simulink model "WESDem_SetPoint"  (R2016b)
settings: configuration reference "CodeGenConfigSet" (kept outside this file)
values from neighbouring files (symbols this model uses):
  EISGov_st3valid_C = Calibration.Parameter    [init_WESDem_SetPoint.m]
  WESDem_dnAcc0_C = Calibration.Parameter    [init_WESDem_SetPoint.m]
  WESDem_dnAcc1_C = Calibration.Parameter    [init_WESDem_SetPoint.m]
  WESDem_dnAcc3_C = Calibration.Parameter    [init_WESDem_SetPoint.m]
  WESDem_dnDecn0_C = Calibration.Parameter    [init_WESDem_SetPoint.m]
  WESDem_dnDecn1_C = Calibration.Parameter    [init_WESDem_SetPoint.m]
  WESDem_dnDecn2_C = Calibration.Parameter    [init_WESDem_SetPoint.m]
  WESDem_nDelta_C = Calibration.Parameter    [init_WESDem_SetPoint.m]
  WESDem_nMin0_C = Calibration.Parameter    [init_WESDem_SetPoint.m]
  WESDem_nMin1_C = Calibration.Parameter    [init_WESDem_SetPoint.m]
  WESDem_nMin2_C = Calibration.Parameter    [init_WESDem_SetPoint.m]
  WESDem_nMin3_C = Calibration.Parameter    [init_WESDem_SetPoint.m]
  WESDem_nMode0_C = Calibration.Parameter    [init_WESDem_SetPoint.m]
  WESDem_nMode1_C = Calibration.Parameter    [init_WESDem_SetPoint.m]
  WESDem_nMode2_C = Calibration.Parameter    [init_WESDem_SetPoint.m]
  WESDem_nMode3_C = Calibration.Parameter    [init_WESDem_SetPoint.m]
  WESDem_nSetPHi0_C = Calibration.Parameter    [init_WESDem_SetPoint.m]
  WESDem_nSetPHi1_C = Calibration.Parameter    [init_WESDem_SetPoint.m]
  WESDem_nSetPHi2_C = Calibration.Parameter    [init_WESDem_SetPoint.m]
  WESDem_nSetPHi3_C = Calibration.Parameter    [init_WESDem_SetPoint.m]
  WESDem_nTipStp_C = Calibration.Parameter    [init_WESDem_SetPoint.m]
  WESDem_rAPPThresFrzI_C = Calibration.Parameter    [init_WESDem_SetPoint.m]
  WESDem_SetPLoTipInRmpSlopeNeg_C = Calibration.Parameter    [init_WESDem_SetPoint.m]
  WESDem_SetPLoTipInRmpSlopePos_C = Calibration.Parameter    [init_WESDem_SetPoint.m]
  WESDem_stASDrfInit_C = Calibration.Parameter    [init_WESDem_SetPoint.m]
  WESDem_stCurr_C = Calibration.Parameter    [init_WESDem_SetPoint.m]
  WESDem_stCurrvalid_C = Calibration.Parameter    [init_WESDem_SetPoint.m]
  WESDem_stMskFrzRls_C = Calibration.Parameter    [init_WESDem_SetPoint.m]
  WESDem_swtTrqHiSel_C = Calibration.Parameter    [init_WESDem_SetPoint.m]
  WESDem_swtTrqLoSel_C = Calibration.Parameter    [init_WESDem_SetPoint.m]
  WESDem_tiPT1_C = Calibration.Parameter    [init_WESDem_SetPoint.m]
  WESDem_tiTrqHiPT1_C = Calibration.Parameter    [init_WESDem_SetPoint.m]
  WESDem_tiTrqLoPT1_C = Calibration.Parameter    [init_WESDem_SetPoint.m]
undefined symbols (not defined in the file or in its folder): CruiseCtl_State_conv, Switch_conv, WESDem_SetPoint_DT, WESDem_State_conv
libraries: CXLib x23, simulink x15
(part 1 of 2)
settings Model: Creator=zhoukai  LastModifiedBy=zhoukai
settings ConfigSetRef: SourceLocation=Base Workspace

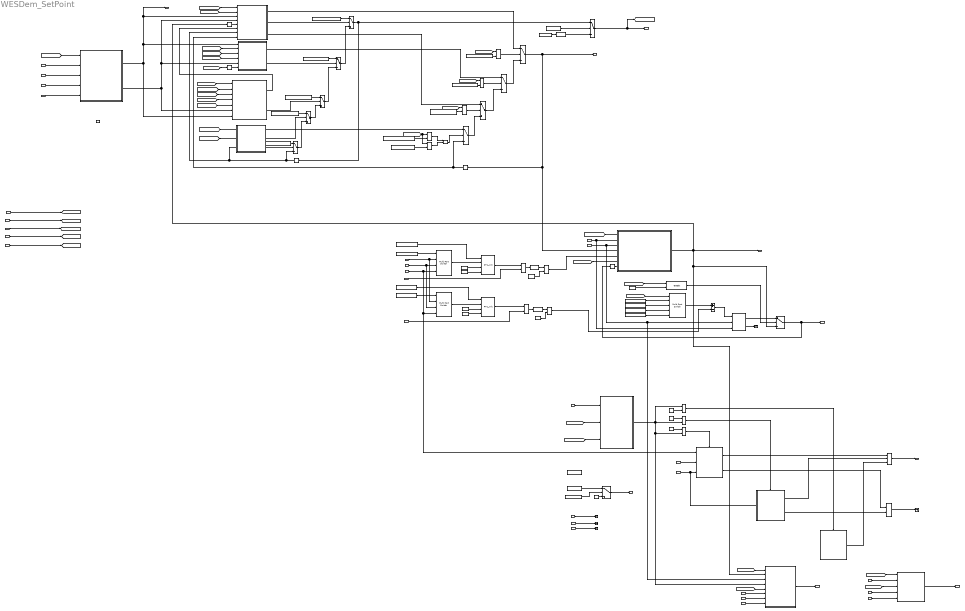
== system WESDem_SetPoint ==
  APP_r : Inport  Tag=%  Description=Acceleration pedal sensor 1 value after fault handling  OutMin=0  OutMax=100  OutDataTypeStr=Accpedal_rate
  CoETS_trqInrSetSlow : Inport  Tag=Nm  Description=Filtered inner torque ( positive torque) desired value (standard signal path) generated out of CoPT_trqDesEng  Port=2  OutMin=-3276  OutMax=3276  OutDataTypeStr=Trq_Nm
  CrCtl_st : Inport  Description=Application parameter for Cruise Control state  Port=3  OutDataTypeStr=Enum: CruiseCtl_State_conv
  DrvDem_swtDrvNGovActv : Inport  Description=Switch to activate DrvDem  Port=4  OutDataTypeStr=Enum: Switch_conv
  GlbDa_stTrqDem : Inport  Description=Contains highest prior function with torque demand  Port=5  OutMin=0  OutMax=4294967295  OutDataTypeStr=State_uint32
  HLSDem_nSetPHi : Inport  Tag=rpm  Description=Maximum engine speed of HLSDem  Port=6  OutMin=0  OutMax=6000  OutDataTypeStr=EngSpeed_rpm
  HLSDem_nSetPLo : Inport  Tag=rpm  Description=Minimum engine speed of HLSDem  Port=7  OutMin=0  OutMax=6000  OutDataTypeStr=EngSpeed_rpm
  MoFPTO_nMax0CalMsgA : Inport  Tag=rpm  Description=MoFPTO_nMaxCalMsgA[0]  Port=8  OutMin=0  OutMax=6000  OutDataTypeStr=EngSpeed_rpm
  MoFPTO_nMax1CalMsgA : Inport  Tag=rpm  Description=MoFPTO_nMaxCalMsgA[1]  Port=9  OutMin=0  OutMax=6000  OutDataTypeStr=EngSpeed_rpm
  MoFPTO_nMax2CalMsgA : Inport  Tag=rpm  Description=MoFPTO_nMaxCalMsgA[2]  Port=10  OutMin=0  OutMax=6000  OutDataTypeStr=EngSpeed_rpm
  MoFPTO_nMax3CalMsgA : Inport  Tag=rpm  Description=MoFPTO_nMaxCalMsgA[3]  Port=11  OutMin=0  OutMax=6000  OutDataTypeStr=EngSpeed_rpm
  PthLead_trqInrCurr : Inport  Tag=Nm  Description=Actual percent engine torque  Port=12  OutMin=-3000  OutMax=3000  OutDataTypeStr=Trq_Nm
  PthLead_trqInrLead : Inport  Tag=Nm  Description=Inner torque lead value  Port=13  OutMin=-3000  OutMax=3000  OutDataTypeStr=Trq_Nm
  PthSet_trqInrSet : Inport  Tag=Nm  Description=Inner torque set value after monitoring limitation  Port=14  OutMin=-3000  OutMax=3276.7  OutDataTypeStr=Trq_Nm
  VehV_v : Inport  Tag=km/h  Description=Vehicle speed  Port=15  OutMin=0  OutMax=250  OutDataTypeStr=VehSpeed_km_h
  WESDem_stCfg : Inport  Description=Configuration of the actual operating mode  Port=16  OutMin=0  OutMax=65535  OutDataTypeStr=State_uint16
  WESDem_stCrCtl : Inport  Description=State control of the working engine speed demand  Port=17  OutMin=0  OutMax=65535  OutDataTypeStr=State_uint16
  WESDem_stMode : Inport  Description=Operating mode of the working engine speed demand  Port=18  OutMin=0  OutMax=255  OutDataTypeStr=State_uint8
  WESDem_stModeChange : Inport  Description=Operating mode change of the working engine speed demand  Port=19  OutMin=0  OutMax=255  OutDataTypeStr=State_uint8
  Epm_nEng : Inport  Tag=rpm  Description=Engine speed  Port=20  OutMin=0  OutMax=6000  OutDataTypeStr=EngSpeed_rpm
  WESDem_facFdbkLo : Inport  Tag=rpm/Nm  Description=Feedback factor for the lower setpoint  Port=21  OutMin=-20  OutMax=20  OutDataTypeStr=FdbkNm2rpm_rpm_Nm
  WESDem_facFdbkHi : Inport  Tag=rpm/Nm  Description=Feedback factor for the higher setpoint  Port=22  OutMin=-20  OutMax=20  OutDataTypeStr=FdbkNm2rpm_rpm_Nm
  WESDem_stStrtBtnSP : Inport  Description=Status of working engine speed setpoint through start button  Port=23  OutMin=0  OutMax=255  OutDataTypeStr=State_uint8
  WESDem_nStrtBtnSP : Inport  Tag=rpm  Description=Working engine speed setpoint through start button  Port=24  OutMin=0  OutMax=6000  OutDataTypeStr=EngSpeed_rpm
  WESDem_stEISGovCfg : Inport  Description=Status of configuration of the EISGov structure  Port=25  OutMin=0  OutMax=255  OutDataTypeStr=State_uint8
  WESDem_vMaxActv : Inport  Tag=km/h  Description=Vehicle speed threshold for activation of the WESDem  Port=26  OutMin=0  OutMax=255  OutDataTypeStr=VehSpeed_km_h
  Asdrf_stInitin : Inport  Description=Status of Initialisation of ASD reference filter  Port=27  OutMin=0  OutMax=255  OutDataTypeStr=State_uint8
  WESDem_stShutOff : Inport  Description=Shut off conditions for the Working engine speed Demand  Port=28  OutMin=0  OutMax=65535  OutDataTypeStr=State_uint16
  function : TriggerPort  TriggerType=function-call  VariantControl=Variant
  ActionToNoInit : Subsystem
  Constant : Constant  Value=WESDem_State_conv.WESDEM_STOFFRAMP  OutDataTypeStr=Inherit: Inherit via back propagation
  Constant1 : Constant  Value=WESDem_swtTrqLoSel_C
  Constant10 : Constant  Value=WESDem_tiTrqHiPT1_C
  Constant11 : Constant  Value=WESDem_State_conv.WESDEM_STNEUTRAL  OutDataTypeStr=Inherit: Inherit via back propagation
  Constant{2..5,12,14,31} (7 alike) : Constant  Value=0  OutDataTypeStr=Inherit: Inherit via back propagation
  Constant13 : Constant  Value=7  OutDataTypeStr=Inherit: Inherit via back propagation
  Constant15 : Constant  Value=WESDem_nSetPHi0_C
  Constant16 : Constant  Value=WESDem_nSetPHi1_C
  Constant17 : Constant  Value=WESDem_nSetPHi2_C
  Constant18 : Constant  Value=WESDem_nSetPHi3_C
  Constant19 : Constant  Value=WESDem_State_conv.WESDEM_STOFF  OutDataTypeStr=Inherit: Inherit via back propagation
  Constant20 : Constant  Value=WESDem_State_conv.WESDEM_STOFFRAMP  OutDataTypeStr=Inherit: Inherit via back propagation
  Constant21 : Constant  Value=WESDem_stCurr_C
  Constant22 : Constant  Value=WESDem_stCurrvalid_C
  Constant23 : Constant  Value=EISGov_st3valid_C
  Constant24 : Constant  Value=WESDem_State_conv.WESDEM_STOFF  OutDataTypeStr=Inherit: Inherit via back propagation
  Constant25 : Constant  Value=WESDem_State_conv.WESDEM_STRESRAMP  OutDataTypeStr=Inherit: Inherit via back propagation
  Constant26 : Constant  Value=WESDem_State_conv.WESDEM_STACCDEC  OutDataTypeStr=Inherit: Inherit via back propagation
  Constant27 : Constant  Value=WESDem_State_conv.WESDEM_STNEUTRAL  OutDataTypeStr=Inherit: Inherit via back propagation
  Constant28 : Constant  Value=0
  Constant29 : Constant
  Constant30 : Constant  Value=2
  Constant6 : Constant  Value=WESDem_State_conv.WESDEM_STRESRAMP  OutDataTypeStr=Inherit: Inherit via back propagation
  Constant7 : Constant  Value=WESDem_swtTrqHiSel_C
  Constant8 : Constant  Value=WESDem_State_conv.WESDEM_STACCDEC  OutDataTypeStr=Inherit: Inherit via back propagation
  Constant9 : Constant  Value=WESDem_tiTrqLoPT1_C
  Data Store Memory : DataStoreMemory  DataStoreName=EISGov_st3  ReadBeforeWriteMsg=warning  WriteAfterWriteMsg=warning  WriteAfterReadMsg=warning  ShowAdditionalParam=off
  Data Store Read : DataStoreRead  DataStoreName=EISGov_st3
  Data Type Conversion : DataTypeConversion
  Data Type Conversion1 : DataTypeConversion
  Data Type Conversion2 : DataTypeConversion
  Delay : Delay  DelayLength=1  InitialCondition=WESDem_State_conv.WESDEM_STOFF
  Delay2 : Delay  DelayLength=1  InitialCondition=0
  Delay3 : Delay  DelayLength=1
  Delay4 : Delay  DelayLength=1
  Delay5 : Delay  DelayLength=1  InitialCondition=WESDem_State_conv.WESDEM_STOFF
  EISGov initialization : Subsystem
  GetBit1 : CXLib/GetBit  dataTypeString=uint16  dataLength=0
      settings: AttributesFormatString=Get bit from %<dataTypeString>
  Interface to the EISGov : Subsystem
  Logical Operator1 : Logic  Operator=OR  AllPortsSameDT=off  OutDataTypeStr=boolean
  Merge : Merge  Inputs=3
  Merge1 : Merge
  MinMax : MinMax  Function=max  Inputs=2
  MinMax1 : MinMax  Function=max  Inputs=2
  Multiport Switch : MultiPortSwitch  DataPortOrder=Zero-based contiguous
  Multiport Switch1 : MultiPortSwitch  DataPortOrder=Zero-based contiguous
  Multiport Switch2 : MultiPortSwitch  DataPortOrder=Zero-based contiguous  Inputs=4
  "Normal operation " : Subsystem  TreatAsAtomicUnit=on
  PT1_Init : CXLib/PT1_Init
  PT1_Init1 : CXLib/PT1_Init
  Product : Product
  Product1 : Product
  Relational Operator{3..10} (8 alike) : RelationalOperator  Operator===  OutDataTypeStr=boolean  RndMeth=Simplest
  Saturation_S1 : CXLib/Saturation_S16
  Subsystem1 : Subsystem
  Subsystem2 : Subsystem
  Subtract1 : Sum  Inputs=+-
  Switch{1..12} (12 alike) : Switch  Criteria=u2 ~= 0
  Terminator{,1..4} (5 alike) : Terminator
  WESDem_OffInit : Subsystem
  WESDem_OnInit : Subsystem
  WESDem_stCrCtl001 : Subsystem
  "WESDem_stCrCtl002 " : Subsystem
  WESDem_stCrCtl004 : Subsystem
  WESDem_stCrCtl007 : Subsystem
  WESDem_nMax : Outport  Tag=rpm  Description=maximum engine speed in selected mode  OutMin=0  OutMax=6000  OutDataTypeStr=EngSpeed_rpm
  WESDem_nSetPHi : Outport  Tag=rpm  Description=Higher setpoint speed interval of WESDem  Port=2  OutMin=0  OutMax=6000  OutDataTypeStr=EngSpeed_rpm
  WESDem_nSetPLo : Outport  Tag=rpm  Description=Lower setpoint speed interval of WESDem  Port=3  OutMin=0  OutMax=6000  OutDataTypeStr=EngSpeed_rpm
  WESDem_stActvReq : Outport  Description=WESDem activation request for EISGov  Port=4  OutMin=0  OutMax=1  OutDataTypeStr=boolean
  WESDem_stCrCtlShutOff : Outport  Description=Shut off of the cruise control  Port=5  OutMin=0  OutMax=1  OutDataTypeStr=boolean
  WESDem_stCurr : Outport  Description=Status of the working engine Speed Control  Port=6  OutDataTypeStr=Enum: WESDem_State_conv
  WESDem_trqReq : Outport  Tag=Nm  Description=Torque intialization request of working engine speed demand  Port=7  OutMin=-3276  OutMax=3276  OutDataTypeStr=Trq_Nm
  WESDem_nPrelimSetP_mp : Outport  Tag=rpm  Description=Engine speed set point before access by external engine speed  Port=8  OutMin=0  OutMax=6000  OutDataTypeStr=EngSpeed_rpm
  EISGov_st3 : Outport  Description=Status information of WESDem client  Port=9  OutMin=0  OutMax=2147483648  OutDataTypeStr=State_uint32
  wires:
  WESDem_stCfg/1 -> [WESDem_stCfg]
  WESDem_stMode/1 -> [WESDem_stMode]
  PthLead_trqInrCurr/1 -> Multiport Switch1/3, Multiport Switch/3
  PthLead_trqInrLead/1 -> Multiport Switch1/2, Multiport Switch/2
  PthSet_trqInrSet/1 -> WESDem_OnInit/1(PthSet_trqInrSet), Multiport Switch1/4, Multiport Switch/4
  Constant1/1 -> Multiport Switch/1
  Multiport Switch/1 -> PT1_Init/2
  Constant9/1 -> PT1_Init/1
  Constant14/1 -> PT1_Init/3
  PT1_Init/1 -> Product/1  "WESDem_trqFdbkLoFlt_mp"
  WESDem_facFdbkLo/1 -> Product/2
  Product/1 -> Data Type Conversion1/1
  Constant3/1 -> MinMax/2
  Constant7/1 -> Multiport Switch1/1
  Multiport Switch1/1 -> PT1_Init1/2
  Constant10/1 -> PT1_Init1/1
  Constant4/1 -> PT1_Init1/3
  PT1_Init1/1 -> Product1/1  "WESDem_trqFdbkHiFlt_mp"
  WESDem_facFdbkHi/1 -> Product1/2
  Product1/1 -> Data Type Conversion/1
  Constant12/1 -> MinMax1/2
  MinMax/1 -> "Normal operation "/5(WESDem_nSetPLoCorVal_mp)  "WESDem_nSetPLoCorVal_mp"
  MinMax1/1 -> Subtract1/2  "WESDem_nSetPHiCorVal_mp"
  [WESDem_stCfg] -> GetBit1/1
  Constant13/1 -> GetBit1/2
  [WESDem_stMode] -> Multiport Switch2/1
  Constant15/1 -> Multiport Switch2/2
  Constant16/1 -> Multiport Switch2/3
  Constant17/1 -> Multiport Switch2/4
  Constant18/1 -> Multiport Switch2/5
  Multiport Switch2/1 -> Subtract1/1
  Subtract1/1 -> Saturation_S1/1
  Saturation_S1/1 -> Switch1/1
  GetBit1/1 -> Switch1/2
  Switch1/1 -> WESDem_nSetPHi/1, Delay4/1  "WESDem_nSetPHi"
  Constant2/1 -> PT1_Init/4
  Constant5/1 -> PT1_Init1/4
  "Normal operation "/1(WESDem_nSetPLo) -> WESDem_nSetPLo/1, Delay3/1, Interface to the EISGov/2(WESDem_nSetPLo), Switch1/3  "WESDem_nSetPLo"
  [WESDem_stMode] -> WESDem_stCrCtl007/3(WESDem_stMode)
  [WESDem_stCfg] -> WESDem_stCrCtl007/1(WESDem_stCfg)
  WESDem_stCrCtl/1 -> [WESDem_stCrCtl]
  [WESDem_stCrCtl] -> WESDem_stCrCtl007/2(WESDem_stCrCtl)
  WESDem_stModeChange/1 -> [WESDem_stModeChange]
  [WESDem_stModeChange] -> WESDem_stCrCtl007/4(WESDem_stModeChange)
  Epm_nEng/1 -> [Epm_nEng]
  [Epm_nEng] -> WESDem_stCrCtl007/5(Epm_nEng)
  Constant20/1 -> Switch5/1
  Switch5/1 -> Switch2/3
  Constant6/1 -> Switch2/1
  Switch2/1 -> Switch3/3
  Constant8/1 -> Switch3/1
  Switch3/1 -> Switch4/3
  Constant11/1 -> Switch4/1
  Constant19/1 -> Switch6/1
  Switch6/1 -> Switch5/3
  WESDem_stCrCtl001/3(STOFF_stENABLE) -> Switch6/2
  WESDem_stCrCtl001/2(STRAMP_stENABLE) -> Switch5/2
  WESDem_stCrCtl007/2(STRESRAMP_stENABLE) -> Switch2/2
  WESDem_stCrCtl004/2(STACCDEC_stENABLE) -> Switch3/2
  WESDem_stCrCtl007/1(WESDem_nTargetSetPRESRAMP) -> "WESDem_stCrCtl002 "/6(WESDem_nTargetSetP_mp)  "WESDem_nTargetSetP_mp"
  Switch4/1 -> Delay/1, Switch11/1
  WESDem_stCrCtl001/1(WESDem_nPrelimSetPSTOFF) -> Switch7/1
  Constant/1 -> Relational Operator3/2
  [WESDem_stCurr] -> Relational Operator4/1, Relational Operator3/1
  Constant24/1 -> Relational Operator4/2
  Relational Operator3/1 -> Logical Operator1/1
  Relational Operator4/1 -> Logical Operator1/2
  Logical Operator1/1 -> Switch7/2
  Switch9/1 -> Switch10/3
  Switch10/1 -> WESDem_nPrelimSetP_mp/1, "Normal operation "/4(WESDem_nPrelimSetP_mp), Delay2/1  "WESDem_nPrelimSetP_mp"
  [WESDem_stCurr] -> Relational Operator5/1
  Constant25/1 -> Relational Operator5/2
  Relational Operator5/1 -> Switch8/2
  [WESDem_stCurr] -> Relational Operator6/1
  Constant26/1 -> Relational Operator6/2
  Relational Operator6/1 -> Switch9/2
  [WESDem_stCurr] -> Relational Operator7/1
  Constant27/1 -> Relational Operator7/2
  Relational Operator7/1 -> Switch10/2
  WESDem_stCrCtl004/1(WESDem_nPrelimSetPACCDEC) -> Switch9/1
  "WESDem_stCrCtl002 "/1(WESDem_nPrelimSetPNEUTRAL) -> Switch10/1
  Constant28/1 -> Relational Operator8/2
  EISGov initialization/1("WESDem_stEISGovInit_mp ") -> Relational Operator8/1, Interface to the EISGov/4(WESDem_stEISGovInit_mp), Relational Operator10/2, Relational Operator9/2  "WESDem_stEISGovInit_mp"
  Constant29/1 -> Relational Operator9/1
  Constant30/1 -> Relational Operator10/1
  Relational Operator8/1 -> ActionToNoInit/Enable
  Relational Operator9/1 -> WESDem_OffInit/Enable
  Relational Operator10/1 -> WESDem_OnInit/Enable
  MoFPTO_nMax0CalMsgA/1 -> Subsystem2/2(MoFPTO_nMax0CalMsgA)
  MoFPTO_nMax1CalMsgA/1 -> Subsystem2/3(MoFPTO_nMax1CalMsgA)
  MoFPTO_nMax2CalMsgA/1 -> Subsystem2/4(MoFPTO_nMax2CalMsgA)
  MoFPTO_nMax3CalMsgA/1 -> Subsystem2/5(MoFPTO_nMax3CalMsgA)
  "WESDem_stCrCtl002 "/2(STNEUTRAL_stENABLE) -> Switch4/2
  Subsystem2/1(WESDem_nMax) -> WESDem_nMax/1, "WESDem_stCrCtl002 "/3(WESDem_nMax), WESDem_stCrCtl004/1(WESDem_nMax), WESDem_stCrCtl007/7(WESDem_nMax)  "WESDem_nMax"
  Subsystem2/2(WESDem_nMin_mp) -> "WESDem_stCrCtl002 "/4(WESDem_nMin_mp), WESDem_stCrCtl004/5(WESDem_nMin_mp), WESDem_stCrCtl007/6(WESDem_nMin_mp)  "WESDem_nMin_mp"
  [WESDem_stCrCtl] -> "WESDem_stCrCtl002 "/1(WESDem_stCrCtl)
  [Epm_nEng] -> "WESDem_stCrCtl002 "/2(Epm_nEng)
  [WESDem_stMode] -> WESDem_stCrCtl004/2(WESDem_stMode)
  [Epm_nEng] -> WESDem_stCrCtl004/3(Epm_nEng)
  [WESDem_stCfg] -> WESDem_stCrCtl004/4(WESDem_stCrCtl)
  [Epm_nEng] -> WESDem_stCrCtl001/2(Epm_nEng)
  [WESDem_stCrCtl] -> WESDem_stCrCtl001/1(WESDem_stCrCtl)
  [WESDem_stMode] -> Subsystem2/1(WESDem_stMode)
  HLSDem_nSetPHi/1 -> Saturation_S1/3, "Normal operation "/2(HLSDem_nSetPHi)
  HLSDem_nSetPLo/1 -> Interface to the EISGov/3(HLSDem_nSetPLo), Saturation_S1/2, "Normal operation "/3(HLSDem_nSetPLo)
  [WESDem_stCfg] -> "Normal operation "/6(WESDem_stCfg)
  Delay4/1 -> "Normal operation "/7(WESDem_nSetPHi)
  Delay3/1 -> "WESDem_stCrCtl002 "/5(WESDem_nSetPLo)
  [WESDem_stCurr] -> Delay5/1
  Delay5/1 -> WESDem_stCrCtl004/6(WESDem_stCurr)
  Delay/1 -> "WESDem_stCrCtl002 "/7(WESDem_stPreCurr), WESDem_stCrCtl001/3(WESDem_stCurr), Switch6/3
  CrCtl_st/1 -> EISGov initialization/1(CrCtl_st)
  [WESDem_stCurr] -> EISGov initialization/2("WESDem_stCurr ")
  [WESDem_stCrCtl] -> EISGov initialization/3(WESDem_stCrCtl)
  CoETS_trqInrSetSlow/1 -> WESDem_OnInit/2(CoETS_trqInrSetSlow)
  Asdrf_stInitin/1 -> WESDem_OffInit/1(Asdrf_stInitin), WESDem_OnInit/3(Asdrf_stInitin)
  WESDem_OnInit/1(WESDem_trqReq) -> Merge/1
  WESDem_OffInit/1(WESDem_trqReq) -> Merge/2
  ActionToNoInit/1(WESDem_trqReq) -> Merge/3
  WESDem_OnInit/2(asdrf_stInitOut) -> Merge1/1
  WESDem_OffInit/2(asdrf_stInitOut) -> Merge1/2
  Merge1/1 -> Terminator/1
  Merge/1 -> WESDem_trqReq/1  "WESDem_trqReq"
  VehV_v/1 -> Subsystem1/4(VehV_v)
  WESDem_vMaxActv/1 -> Subsystem1/5(WESDem_vMaxActv)
  WESDem_stShutOff/1 -> Subsystem1/2(WESDem_stShutOff)
  [WESDem_stCfg] -> Subsystem1/1(WESDem_stCfg)
  APP_r/1 -> Interface to the EISGov/6(APP_r)
  DrvDem_swtDrvNGovActv/1 -> Interface to the EISGov/7(DrvDem_swtDrvNGovActv)
  GlbDa_stTrqDem/1 -> Interface to the EISGov/8("GlbDa_stTrqDem ")
  Subsystem1/1(WESDem_stCrCtlShutOff) -> WESDem_stCrCtlShutOff/1  "WESDem_stCrCtlShutOff"
  Interface to the EISGov/1(WESDem_stActvReq) -> WESDem_stActvReq/1  "WESDem_stActvReq"
  [Epm_nEng] -> Interface to the EISGov/5(Epm_nEng)
  [WESDem_stCurr] -> Interface to the EISGov/1("WESDem_stCurr ")
  [WESDem_stCurr] -> Subsystem1/3("WESDem_stCurr ")
  WESDem_stEISGovCfg/1 -> Terminator1/1
  WESDem_stStrtBtnSP/1 -> Terminator2/1
  WESDem_nStrtBtnSP/1 -> Terminator3/1
  Data Type Conversion/1 -> MinMax1/1
  Data Type Conversion1/1 -> MinMax/1
  Saturation_S1/2 -> Terminator4/1
  [WESDem_stCurr] -> "Normal operation "/1(WESDem_stCurr)
  Delay2/1 -> Switch7/3, "WESDem_stCrCtl002 "/8(WESDem_nPrelimSetPTipSt)
  Switch7/1 -> Switch8/3
  Switch8/1 -> Switch9/3
  "WESDem_stCrCtl002 "/3(WESDem_nPrelimSetPRESRAMP) -> Switch8/1
  Switch11/1 -> [WESDem_stCurr], WESDem_stCurr/1  "WESDem_stCurr"
  Constant21/1 -> Data Type Conversion2/1
  Data Type Conversion2/1 -> Switch11/3
  Constant22/1 -> Switch11/2
  Switch12/1 -> EISGov_st3/1  "EISGov_st3"
  Data Store Read/1 -> Switch12/1
  Constant23/1 -> Switch12/2
  Constant31/1 -> Switch12/3

== system WESDem_SetPoint/ActionToNoInit ==
  Enable : EnablePort
  Bit Clear : simulink/Logic and Bit Operations/Bit Clear  iBit=3
  Bit Clear1 : simulink/Logic and Bit Operations/Bit Clear  iBit=3
  Constant3 : Constant  Value=0  OutDataTypeStr=Inherit: Inherit via back propagation
  Data Store Read3 : DataStoreRead  DataStoreName=EISGov_st3
  Data Store Write2 : DataStoreWrite  DataStoreName=EISGov_st3
  WESDem_trqReq : Outport  Tag=Nm  Description=Torque intialization request of working engine speed demand  OutMin=-3276  OutMax=3276  OutDataTypeStr=Trq_Nm
  wires:
  Data Store Read3/1 -> Bit Clear/1
  Bit Clear/1 -> Bit Clear1/1
  Bit Clear1/1 -> Data Store Write2/1
  Constant3/1 -> WESDem_trqReq/1

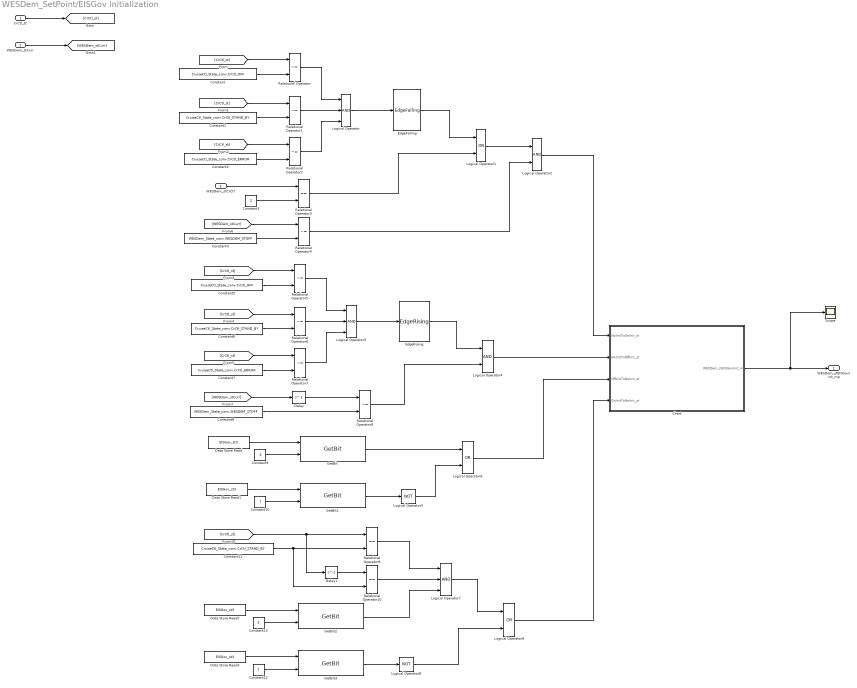
== system WESDem_SetPoint/EISGov initialization ==
  CrCtl_st : Inport  Description=Application parameter for Cruise Control state
  "WESDem_stCurr " : Inport  Description=Application parameter for Cruise Control state  Port=2  OutDataTypeStr=Enum: WESDem_State_conv
  WESDem_stCrCtl : Inport  Description=State control of the working engine speed demand  Port=3  OutMin=0  OutMax=65535  OutDataTypeStr=State_uint16
  Chart : Stateflow chart  TreatAsAtomicUnit=on
  Constant : Constant  Value=CruiseCtl_State_conv.CrCtl_OFF  OutDataTypeStr=Inherit: Inherit via back propagation
  Constant1 : Constant  Value=CruiseCtl_State_conv.CrCtl_STAND_BY  OutDataTypeStr=Inherit: Inherit via back propagation
  Constant10 : Constant  Value=7  OutDataTypeStr=Inherit: Inherit via back propagation
  Constant11 : Constant  Value=CruiseCtl_State_conv.CrCtl_STAND_BY  OutDataTypeStr=Inherit: Inherit via back propagation
  Constant12 : Constant  Value=7  OutDataTypeStr=Inherit: Inherit via back propagation
  Constant13 : Constant  Value=3  OutDataTypeStr=Inherit: Inherit via back propagation
  Constant2 : Constant  Value=CruiseCtl_State_conv.CrCtl_ERROR  OutDataTypeStr=Inherit: Inherit via back propagation
  Constant3 : Constant  Value=2  OutDataTypeStr=Inherit: Inherit via back propagation
  Constant4 : Constant  Value=WESDem_State_conv.WESDEM_STOFF  OutDataTypeStr=Inherit: Inherit via back propagation
  Constant5 : Constant  Value=CruiseCtl_State_conv.CrCtl_OFF  OutDataTypeStr=Inherit: Inherit via back propagation
  Constant6 : Constant  Value=CruiseCtl_State_conv.CrCtl_STAND_BY
  Constant7 : Constant  Value=CruiseCtl_State_conv.CrCtl_ERROR  OutDataTypeStr=Inherit: Inherit via back propagation
  Constant8 : Constant  Value=WESDem_State_conv.WESDEM_STOFF  OutDataTypeStr=Inherit: Inherit via back propagation
  Constant9 : Constant  Value=3  OutDataTypeStr=Inherit: Inherit via back propagation
  Data Store Read{,1..3} (4 alike) : DataStoreRead  DataStoreName=EISGov_st3
  Delay : Delay  DelayLength=1  InitialCondition=WESDem_State_conv.WESDEM_STNEUTRAL
  Delay1 : Delay  DelayLength=1  InitialCondition=CruiseCtl_State_conv.CrCtl_OFF
  EdgeFalling : CXLib/EdgeFalling
  EdgeRising : CXLib/EdgeRising
  GetBit{,1..3} (4 alike) : CXLib/GetBit  dataTypeString=uint32  dataLength=0
      settings: AttributesFormatString=Get bit from %<dataTypeString>
  Logical Operator : Logic  Inputs=3  AllPortsSameDT=off  OutDataTypeStr=boolean
  Logical Operator1 : Logic  Operator=OR  AllPortsSameDT=off  OutDataTypeStr=boolean
  Logical Operator2 : Logic  AllPortsSameDT=off  OutDataTypeStr=boolean
  Logical Operator3 : Logic  Inputs=3  AllPortsSameDT=off  OutDataTypeStr=boolean
  Logical Operator4 : Logic  AllPortsSameDT=off  OutDataTypeStr=boolean
  Logical Operator5 : Logic  Operator=NOT  AllPortsSameDT=off  OutDataTypeStr=boolean
  Logical Operator6 : Logic  Operator=OR  AllPortsSameDT=off  OutDataTypeStr=boolean
  Logical Operator7 : Logic  Inputs=3  AllPortsSameDT=off  OutDataTypeStr=boolean
  Logical Operator8 : Logic  Operator=NOT  AllPortsSameDT=off  OutDataTypeStr=boolean
  Logical Operator9 : Logic  Operator=OR  AllPortsSameDT=off  OutDataTypeStr=boolean
  Relational Operator{,1..2,4..8} (8 alike) : RelationalOperator  Operator=~=  OutDataTypeStr=boolean  RndMeth=Simplest
  Relational Operator10 : RelationalOperator  Operator===  OutDataTypeStr=boolean  RndMeth=Simplest
  Relational Operator3 : RelationalOperator  Operator===  OutDataTypeStr=boolean  RndMeth=Simplest
  Relational Operator9 : RelationalOperator  Operator===  OutDataTypeStr=boolean  RndMeth=Simplest
  Scope : Scope
  "WESDem_stEISGovInit_mp " : Outport
  wires:
  CrCtl_st/1 -> [CrCtl_st]
  [CrCtl_st] -> Relational Operator/1
  Constant/1 -> Relational Operator/2
  [CrCtl_st] -> Relational Operator1/1
  Constant1/1 -> Relational Operator1/2
  [CrCtl_st] -> Relational Operator2/1
  Constant2/1 -> Relational Operator2/2
  Relational Operator1/1 -> Logical Operator/2
  Relational Operator/1 -> Logical Operator/1
  Relational Operator2/1 -> Logical Operator/3
  Logical Operator/1 -> EdgeFalling/1
  WESDem_stCrCtl/1 -> Relational Operator3/1
  Constant3/1 -> Relational Operator3/2
  EdgeFalling/1 -> Logical Operator1/1
  Relational Operator3/1 -> Logical Operator1/2
  Constant4/1 -> Relational Operator4/2
  Logical Operator1/1 -> Logical Operator2/1
  Relational Operator4/1 -> Logical Operator2/2
  [CrCtl_st] -> Relational Operator5/1
  Constant5/1 -> Relational Operator5/2
  [CrCtl_st] -> Relational Operator6/1
  Constant6/1 -> Relational Operator6/2
  [CrCtl_st] -> Relational Operator7/1
  Constant7/1 -> Relational Operator7/2
  Relational Operator6/1 -> Logical Operator3/2
  Relational Operator5/1 -> Logical Operator3/1
  Relational Operator7/1 -> Logical Operator3/3
  Logical Operator3/1 -> EdgeRising/1
  [WESDem_stCurr] -> Delay/1
  Constant8/1 -> Relational Operator8/2
  Relational Operator8/1 -> Logical Operator4/2
  EdgeRising/1 -> Logical Operator4/1
  "WESDem_stCurr "/1 -> [WESDem_stCurr]
  [WESDem_stCurr] -> Relational Operator4/1
  Delay/1 -> Relational Operator8/1
  Data Store Read/1 -> GetBit/1
  Constant9/1 -> GetBit/2
  Constant10/1 -> GetBit1/2
  GetBit1/1 -> Logical Operator5/1
  GetBit/1 -> Logical Operator6/1
  Logical Operator5/1 -> Logical Operator6/2
  [CrCtl_st] -> Delay1/1, Relational Operator9/1
  Constant11/1 -> Relational Operator10/2, Relational Operator9/2
  Delay1/1 -> Relational Operator10/1
  Relational Operator10/1 -> Logical Operator7/2
  Relational Operator9/1 -> Logical Operator7/1
  Data Store Read2/1 -> GetBit2/1
  Constant13/1 -> GetBit2/2
  Data Store Read3/1 -> GetBit3/1
  Constant12/1 -> GetBit3/2
  GetBit3/1 -> Logical Operator8/1
  GetBit2/1 -> Logical Operator7/3
  Logical Operator8/1 -> Logical Operator9/2
  Logical Operator7/1 -> Logical Operator9/1
  Logical Operator2/1 -> Chart/1(NoInitToOnInit_st)
  Logical Operator4/1 -> Chart/2(NoInitToOffInit_st)
  Logical Operator6/1 -> Chart/3(OffInitToNoInit_st)
  Logical Operator9/1 -> Chart/4(OnInitToNoInit_st)
  Chart/1(WESDem_stEISGovInit_mp) -> Scope/1, "WESDem_stEISGovInit_mp "/1
  Data Store Read1/1 -> GetBit1/1

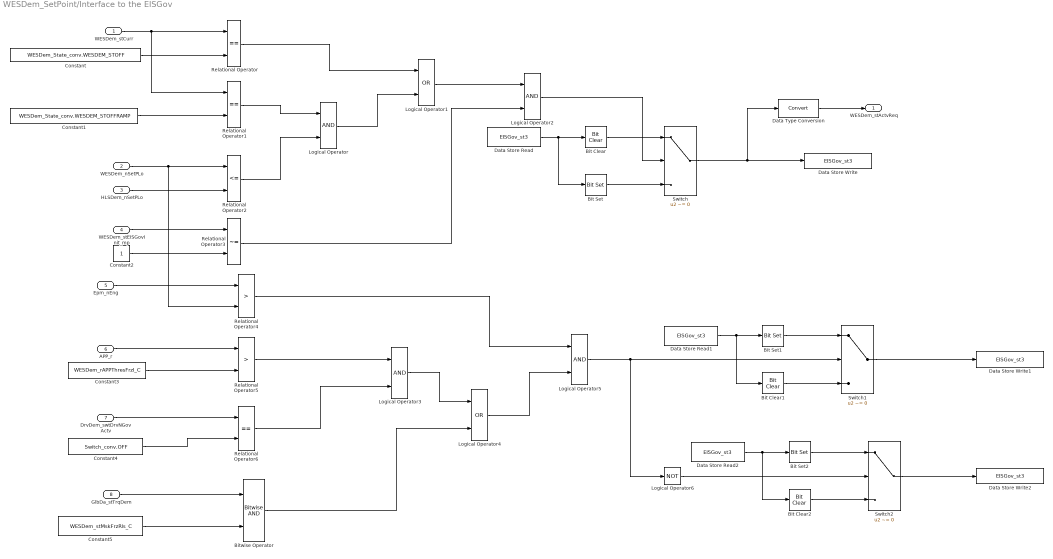
== system WESDem_SetPoint/Interface to the EISGov ==
  "WESDem_stCurr " : Inport  Description=Configuration of the actual operating mode  OutDataTypeStr=Enum: WESDem_State_conv
  WESDem_nSetPLo : Inport  Tag=rpm  Description=Minimum engine speed of HLSDem  Port=2  OutMin=0  OutMax=6000  OutDataTypeStr=EngSpeed_rpm
  HLSDem_nSetPLo : Inport  Tag=rpm  Description=Minimum engine speed of HLSDem  Port=3  OutMin=0  OutMax=6000  OutDataTypeStr=EngSpeed_rpm
  WESDem_stEISGovInit_mp : Inport  Port=4
  Epm_nEng : Inport  Tag=rpm  Description=Engine speed  Port=5  OutMin=0  OutMax=6000  OutDataTypeStr=EngSpeed_rpm
  APP_r : Inport  Port=6
  DrvDem_swtDrvNGovActv : Inport  Description=Switch to activate DrvDem  Port=7  OutDataTypeStr=Enum: Switch_conv
  "GlbDa_stTrqDem " : Inport  Port=8
  Bit Clear : simulink/Logic and Bit Operations/Bit Clear  iBit=7
  Bit Clear1 : simulink/Logic and Bit Operations/Bit Clear  iBit=0
  Bit Clear2 : simulink/Logic and Bit Operations/Bit Clear  iBit=1
  Bit Set : simulink/Logic and Bit Operations/Bit Set  iBit=7
  Bit Set1 : simulink/Logic and Bit Operations/Bit Set  iBit=0
  Bit Set2 : simulink/Logic and Bit Operations/Bit Set  iBit=1
  Bitwise Operator : simulink/Logic and Bit Operations/Bitwise Operator  logicop=AND  UseBitMask=off  NumInputPorts=2  BitMask=bin2dec('11011001')  BitMaskRealWorld=Stored Integer
  Constant : Constant  Value=WESDem_State_conv.WESDEM_STOFF  OutDataTypeStr=Inherit: Inherit via back propagation
  Constant1 : Constant  Value=WESDem_State_conv.WESDEM_STOFFRAMP  OutDataTypeStr=Inherit: Inherit via back propagation
  Constant2 : Constant  OutDataTypeStr=Inherit: Inherit via back propagation
  Constant3 : Constant  Value=WESDem_rAPPThresFrzI_C
  Constant4 : Constant  Value=Switch_conv.OFF  OutDataTypeStr=Enum: Switch_conv
  Constant5 : Constant  Value=WESDem_stMskFrzRls_C
  Data Store Read : DataStoreRead  DataStoreName=EISGov_st3
  Data Store Read1 : DataStoreRead  DataStoreName=EISGov_st3
  Data Store Read2 : DataStoreRead  DataStoreName=EISGov_st3
  Data Store Write : DataStoreWrite  DataStoreName=EISGov_st3
  Data Store Write1 : DataStoreWrite  DataStoreName=EISGov_st3
  Data Store Write2 : DataStoreWrite  DataStoreName=EISGov_st3
  Data Type Conversion : DataTypeConversion
  Logical Operator{,2..3,5} (4 alike) : Logic  AllPortsSameDT=off  OutDataTypeStr=boolean
  Logical Operator1 : Logic  Operator=OR  AllPortsSameDT=off  OutDataTypeStr=boolean
  Logical Operator4 : Logic  Operator=OR  AllPortsSameDT=off  OutDataTypeStr=boolean
  Logical Operator6 : Logic  Operator=NOT  AllPortsSameDT=off  OutDataTypeStr=boolean
  Relational Operator : RelationalOperator  Operator===  OutDataTypeStr=boolean  RndMeth=Simplest
  Relational Operator1 : RelationalOperator  Operator===  OutDataTypeStr=boolean  RndMeth=Simplest
  Relational Operator2 : RelationalOperator  Operator=<=  OutDataTypeStr=boolean  RndMeth=Simplest
  Relational Operator3 : RelationalOperator  Operator=~=  OutDataTypeStr=boolean  RndMeth=Simplest
  Relational Operator4 : RelationalOperator  Operator=>  OutDataTypeStr=boolean  RndMeth=Simplest
  Relational Operator5 : RelationalOperator  Operator=>  OutDataTypeStr=boolean  RndMeth=Simplest
  Relational Operator6 : RelationalOperator  Operator===  OutDataTypeStr=boolean  RndMeth=Simplest
  Switch : Switch  Criteria=u2 ~= 0
  Switch1 : Switch  Criteria=u2 ~= 0
  Switch2 : Switch  Criteria=u2 ~= 0
  WESDem_stActvReq : Outport  Description=WESDem activation request for EISGov  OutMin=0  OutMax=1  OutDataTypeStr=boolean
  wires:
  Constant/1 -> Relational Operator/2
  "WESDem_stCurr "/1 -> Relational Operator1/1, Relational Operator/1
  Constant1/1 -> Relational Operator1/2
  HLSDem_nSetPLo/1 -> Relational Operator2/2
  Relational Operator1/1 -> Logical Operator/1
  Relational Operator2/1 -> Logical Operator/2
  Relational Operator/1 -> Logical Operator1/1
  Logical Operator/1 -> Logical Operator1/2
  WESDem_stEISGovInit_mp/1 -> Relational Operator3/1
  Constant2/1 -> Relational Operator3/2
  Logical Operator1/1 -> Logical Operator2/1
  Relational Operator3/1 -> Logical Operator2/2
  Switch/1 -> Data Store Write/1, Data Type Conversion/1
  Logical Operator2/1 -> Switch/2
  Bit Clear/1 -> Switch/1
  Bit Set/1 -> Switch/3
  Epm_nEng/1 -> Relational Operator4/1
  WESDem_nSetPLo/1 -> Relational Operator4/2, Relational Operator2/1
  APP_r/1 -> Relational Operator5/1
  Constant3/1 -> Relational Operator5/2
  DrvDem_swtDrvNGovActv/1 -> Relational Operator6/1
  Constant4/1 -> Relational Operator6/2
  Relational Operator5/1 -> Logical Operator3/1
  Relational Operator6/1 -> Logical Operator3/2
  "GlbDa_stTrqDem "/1 -> Bitwise Operator/1
  Constant5/1 -> Bitwise Operator/2
  Bitwise Operator/1 -> Logical Operator4/2
  Logical Operator3/1 -> Logical Operator4/1
  Relational Operator4/1 -> Logical Operator5/1
  Logical Operator4/1 -> Logical Operator5/2
  Logical Operator5/1 -> Logical Operator6/1, Switch1/2
  Data Store Read/1 -> Bit Set/1, Bit Clear/1
  Switch1/1 -> Data Store Write1/1
  Data Store Read1/1 -> Bit Clear1/1, Bit Set1/1
  Bit Set1/1 -> Switch1/1
  Bit Clear1/1 -> Switch1/3
  Switch2/1 -> Data Store Write2/1
  Data Store Read2/1 -> Bit Clear2/1, Bit Set2/1
  Bit Set2/1 -> Switch2/1
  Bit Clear2/1 -> Switch2/3
  Logical Operator6/1 -> Switch2/2
  Data Type Conversion/1 -> WESDem_stActvReq/1

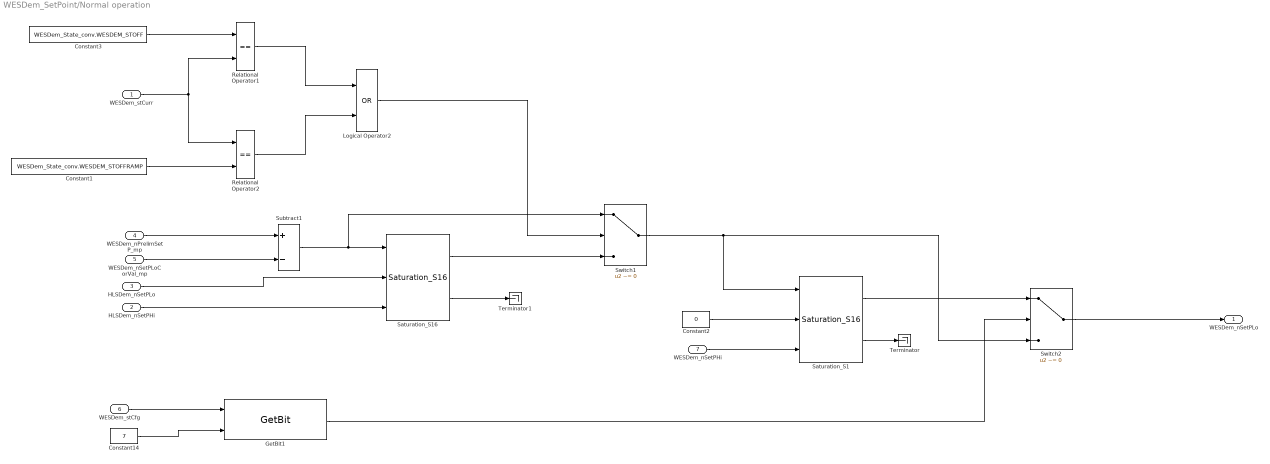
== system WESDem_SetPoint/Normal operation  ==
  WESDem_stCurr : Inport  Description=Configuration of the actual operating mode  OutDataTypeStr=Enum: WESDem_State_conv
  HLSDem_nSetPHi : Inport  Tag=rpm  Description=Maximum engine speed of HLSDem  Port=2  OutMin=0  OutMax=6000  OutDataTypeStr=EngSpeed_rpm
  HLSDem_nSetPLo : Inport  Tag=rpm  Description=Minimum engine speed of HLSDem  Port=3  OutMin=0  OutMax=6000  OutDataTypeStr=EngSpeed_rpm
  WESDem_nPrelimSetP_mp : Inport  Tag=rpm  Description=Maximum engine speed of HLSDem  Port=4  OutMin=0  OutMax=6000  OutDataTypeStr=EngSpeed_rpm
  WESDem_nSetPLoCorVal_mp : Inport  Tag=rpm  Description=Maximum engine speed of HLSDem  Port=5  OutMin=0  OutMax=6000  OutDataTypeStr=EngSpeed_rpm
  WESDem_stCfg : Inport  Description=Configuration of the actual operating mode  Port=6  OutMin=0  OutMax=65535  OutDataTypeStr=State_uint16
  WESDem_nSetPHi : Inport  Tag=rpm  Description=Engine speed  Port=7  OutMin=0  OutMax=6000  OutDataTypeStr=EngSpeed_rpm
  Constant1 : Constant  Value=WESDem_State_conv.WESDEM_STOFFRAMP
  Constant14 : Constant  Value=7  OutDataTypeStr=Inherit: Inherit via back propagation
  Constant2 : Constant  Value=0  OutDataTypeStr=Inherit: Inherit via back propagation
  Constant3 : Constant  Value=WESDem_State_conv.WESDEM_STOFF
  GetBit1 : CXLib/GetBit  dataTypeString=uint16  dataLength=0
      settings: AttributesFormatString=Get bit from %<dataTypeString>
  Logical Operator2 : Logic  Operator=OR  AllPortsSameDT=off  OutDataTypeStr=boolean
  Relational Operator1 : RelationalOperator  Operator===  OutDataTypeStr=boolean  RndMeth=Simplest
  Relational Operator2 : RelationalOperator  Operator===  OutDataTypeStr=boolean  RndMeth=Simplest
  Saturation_S1 : CXLib/Saturation_S16
  Saturation_S16 : CXLib/Saturation_S16
  Subtract1 : Sum  Inputs=+-
  Switch1 : Switch  Criteria=u2 ~= 0
  Switch2 : Switch  Criteria=u2 ~= 0
  Terminator : Terminator
  Terminator1 : Terminator
  WESDem_nSetPLo : Outport  Tag=rpm  Description=Lower setpoint speed interval of WESDem  OutMin=0  OutMax=6000  OutDataTypeStr=EngSpeed_rpm
  wires:
  Constant3/1 -> Relational Operator1/1
  Constant1/1 -> Relational Operator2/2
  WESDem_stCurr/1 -> Relational Operator2/1, Relational Operator1/2
  Relational Operator1/1 -> Logical Operator2/1
  Relational Operator2/1 -> Logical Operator2/2
  WESDem_nPrelimSetP_mp/1 -> Subtract1/1
  WESDem_nSetPLoCorVal_mp/1 -> Subtract1/2
  Subtract1/1 -> Switch1/1, Saturation_S16/1
  HLSDem_nSetPLo/1 -> Saturation_S16/2
  HLSDem_nSetPHi/1 -> Saturation_S16/3
  Logical Operator2/1 -> Switch1/2
  Saturation_S16/1 -> Switch1/3
  WESDem_stCfg/1 -> GetBit1/1
  Constant14/1 -> GetBit1/2
  Switch1/1 -> Switch2/3, Saturation_S1/1
  Constant2/1 -> Saturation_S1/2
  WESDem_nSetPHi/1 -> Saturation_S1/3
  Saturation_S1/1 -> Switch2/1
  GetBit1/1 -> Switch2/2
  Switch2/1 -> WESDem_nSetPLo/1
  Saturation_S1/2 -> Terminator/1
  Saturation_S16/2 -> Terminator1/1

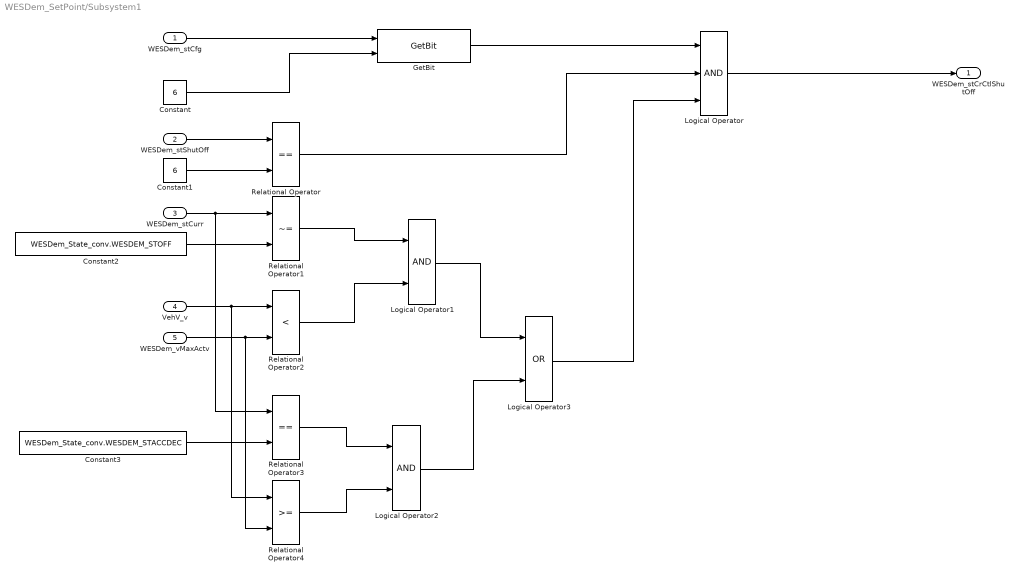
== system WESDem_SetPoint/Subsystem1 ==
  WESDem_stCfg : Inport  Description=Configuration of the actual operating mode  OutMin=0  OutMax=65535  OutDataTypeStr=State_uint16
  WESDem_stShutOff : Inport  Description=Shut off conditions for the Working engine speed Demand  Port=2  OutMin=0  OutMax=65535  OutDataTypeStr=State_uint16
  "WESDem_stCurr " : Inport  Description=Configuration of the actual operating mode  Port=3  OutDataTypeStr=Enum: WESDem_State_conv
  VehV_v : Inport  Tag=km/h  Description=Vehicle speed  Port=4  OutMin=0  OutMax=250  OutDataTypeStr=VehSpeed_km_h
  WESDem_vMaxActv : Inport  Tag=km/h  Description=Vehicle speed threshold for activation of the WESDem  Port=5  OutMin=0  OutMax=255  OutDataTypeStr=VehSpeed_km_h
  Constant : Constant  Value=6  OutDataTypeStr=Inherit: Inherit via back propagation
  Constant1 : Constant  Value=6  OutDataTypeStr=Inherit: Inherit via back propagation
  Constant2 : Constant  Value=WESDem_State_conv.WESDEM_STOFF  OutDataTypeStr=Inherit: Inherit via back propagation
  Constant3 : Constant  Value=WESDem_State_conv.WESDEM_STACCDEC  OutDataTypeStr=Inherit: Inherit via back propagation
  GetBit : CXLib/GetBit  dataTypeString=uint16  dataLength=0
      settings: AttributesFormatString=Get bit from %<dataTypeString>
  Logical Operator : Logic  Inputs=3  AllPortsSameDT=off  OutDataTypeStr=boolean
  Logical Operator1 : Logic  AllPortsSameDT=off  OutDataTypeStr=boolean
  Logical Operator2 : Logic  AllPortsSameDT=off  OutDataTypeStr=boolean
  Logical Operator3 : Logic  Operator=OR  AllPortsSameDT=off  OutDataTypeStr=boolean
  Relational Operator : RelationalOperator  Operator===  OutDataTypeStr=boolean  RndMeth=Simplest
  Relational Operator1 : RelationalOperator  Operator=~=  OutDataTypeStr=boolean  RndMeth=Simplest
  Relational Operator2 : RelationalOperator  Operator=<  OutDataTypeStr=boolean  RndMeth=Simplest
  Relational Operator3 : RelationalOperator  Operator===  OutDataTypeStr=boolean  RndMeth=Simplest
  Relational Operator4 : RelationalOperator  OutDataTypeStr=boolean  RndMeth=Simplest
  WESDem_stCrCtlShutOff : Outport  Description=Shut off of the cruise control  OutMin=0  OutMax=1  OutDataTypeStr=boolean
  wires:
  WESDem_stCfg/1 -> GetBit/1
  Constant/1 -> GetBit/2
  WESDem_stShutOff/1 -> Relational Operator/1
  Constant1/1 -> Relational Operator/2
  "WESDem_stCurr "/1 -> Relational Operator3/1, Relational Operator1/1
  Constant2/1 -> Relational Operator1/2
  GetBit/1 -> Logical Operator/1
  Relational Operator/1 -> Logical Operator/2
  VehV_v/1 -> Relational Operator4/1, Relational Operator2/1
  WESDem_vMaxActv/1 -> Relational Operator4/2, Relational Operator2/2
  Relational Operator1/1 -> Logical Operator1/1
  Relational Operator2/1 -> Logical Operator1/2
  Constant3/1 -> Relational Operator3/2
  Relational Operator3/1 -> Logical Operator2/1
  Relational Operator4/1 -> Logical Operator2/2
  Logical Operator2/1 -> Logical Operator3/2
  Logical Operator1/1 -> Logical Operator3/1
  Logical Operator3/1 -> Logical Operator/3
  Logical Operator/1 -> WESDem_stCrCtlShutOff/1

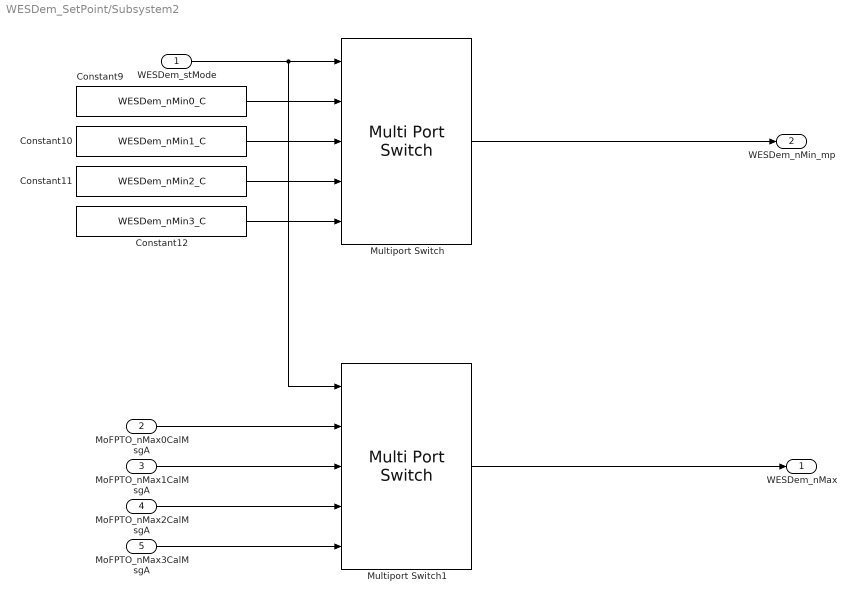
== system WESDem_SetPoint/Subsystem2 ==
  WESDem_stMode : Inport  Description=Operating mode of the working engine speed demand  OutMin=0  OutMax=255  OutDataTypeStr=State_uint8
  MoFPTO_nMax0CalMsgA : Inport  Tag=rpm  Description=MoFPTO_nMaxCalMsgA[0]  Port=2  OutMin=0  OutMax=6000  OutDataTypeStr=EngSpeed_rpm
  MoFPTO_nMax1CalMsgA : Inport  Tag=rpm  Description=MoFPTO_nMaxCalMsgA[1]  Port=3  OutMin=0  OutMax=6000  OutDataTypeStr=EngSpeed_rpm
  MoFPTO_nMax2CalMsgA : Inport  Tag=rpm  Description=MoFPTO_nMaxCalMsgA[2]  Port=4  OutMin=0  OutMax=6000  OutDataTypeStr=EngSpeed_rpm
  MoFPTO_nMax3CalMsgA : Inport  Tag=rpm  Description=MoFPTO_nMaxCalMsgA[3]  Port=5  OutMin=0  OutMax=6000  OutDataTypeStr=EngSpeed_rpm
  Constant10 : Constant  Value=WESDem_nMin1_C
  Constant11 : Constant  Value=WESDem_nMin2_C
  Constant12 : Constant  Value=WESDem_nMin3_C
  Constant9 : Constant  Value=WESDem_nMin0_C
  Multiport Switch : MultiPortSwitch  DataPortOrder=Zero-based contiguous  Inputs=4
  Multiport Switch1 : MultiPortSwitch  DataPortOrder=Zero-based contiguous  Inputs=4
  WESDem_nMax : Outport  Tag=rpm  Description=maximum engine speed in selected mode  OutMin=0  OutMax=6000  OutDataTypeStr=EngSpeed_rpm
  WESDem_nMin_mp : Outport  Tag=rpm  Description=maximum engine speed in selected mode  Port=2  OutMin=0  OutMax=6000  OutDataTypeStr=EngSpeed_rpm
  wires:
  Constant9/1 -> Multiport Switch/2
  Constant10/1 -> Multiport Switch/3
  Constant11/1 -> Multiport Switch/4
  Constant12/1 -> Multiport Switch/5
  MoFPTO_nMax0CalMsgA/1 -> Multiport Switch1/2
  MoFPTO_nMax3CalMsgA/1 -> Multiport Switch1/5
  MoFPTO_nMax1CalMsgA/1 -> Multiport Switch1/3
  WESDem_stMode/1 -> Multiport Switch1/1, Multiport Switch/1
  MoFPTO_nMax2CalMsgA/1 -> Multiport Switch1/4
  Multiport Switch1/1 -> WESDem_nMax/1
  Multiport Switch/1 -> WESDem_nMin_mp/1

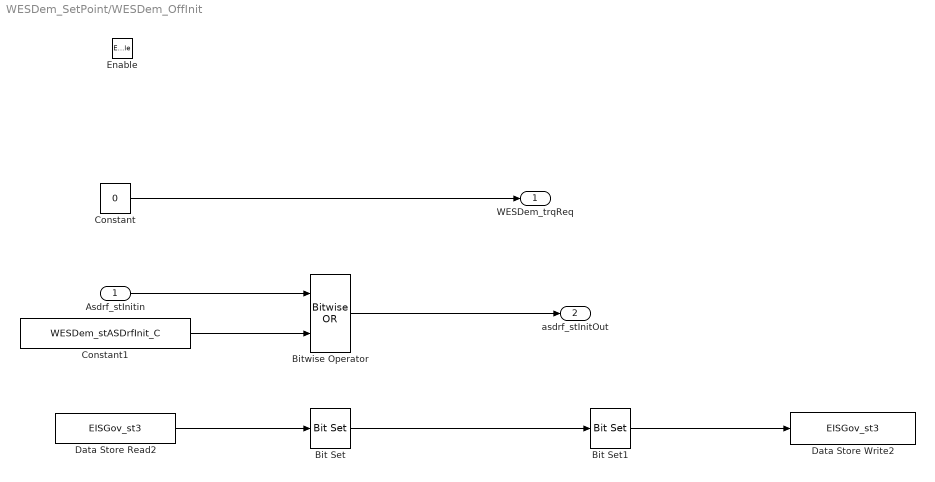
== system WESDem_SetPoint/WESDem_OffInit ==
  Asdrf_stInitin : Inport  Description=Status of Initialisation of ASD reference filter  OutMin=0  OutMax=255  OutDataTypeStr=State_uint8
  Enable : EnablePort
  Bit Set : simulink/Logic and Bit Operations/Bit Set  iBit=2
  Bit Set1 : simulink/Logic and Bit Operations/Bit Set  iBit=3
  Bitwise Operator : simulink/Logic and Bit Operations/Bitwise Operator  logicop=OR  UseBitMask=off  NumInputPorts=2  BitMask=bin2dec('11011001')  BitMaskRealWorld=Stored Integer
  Constant : Constant  Value=0  OutDataTypeStr=Inherit: Inherit via back propagation
  Constant1 : Constant  Value=WESDem_stASDrfInit_C  OutMin=0  OutMax=255
  Data Store Read2 : DataStoreRead  DataStoreName=EISGov_st3
  Data Store Write2 : DataStoreWrite  DataStoreName=EISGov_st3
  WESDem_trqReq : Outport  Tag=Nm  Description=Torque intialization request of working engine speed demand  OutMin=-3276  OutMax=3276  OutDataTypeStr=Trq_Nm
  asdrf_stInitOut : Outport  Port=2  OutMin=0  OutMax=255
  wires:
  Constant/1 -> WESDem_trqReq/1
  Constant1/1 -> Bitwise Operator/2
  Asdrf_stInitin/1 -> Bitwise Operator/1
  Bitwise Operator/1 -> asdrf_stInitOut/1
  Data Store Read2/1 -> Bit Set/1
  Bit Set/1 -> Bit Set1/1
  Bit Set1/1 -> Data Store Write2/1

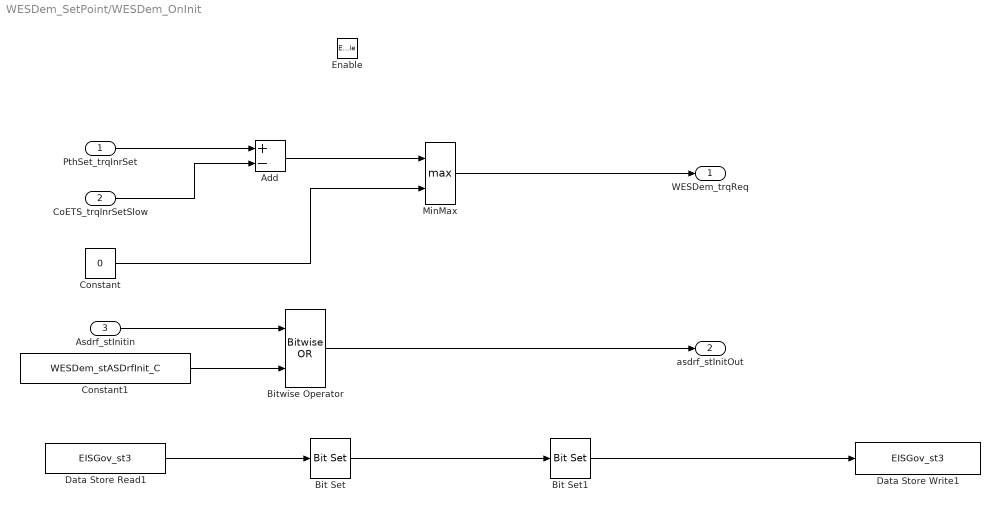
== system WESDem_SetPoint/WESDem_OnInit ==
  PthSet_trqInrSet : Inport  Tag=Nm  Description=Inner torque set value after monitoring limitation  OutMin=-3000  OutMax=3276.7  OutDataTypeStr=Trq_Nm
  CoETS_trqInrSetSlow : Inport  Tag=Nm  Description=Filtered inner torque ( positive torque) desired value (standard signal path) generated out of CoPT_trqDesEng  Port=2  OutMin=-3276  OutMax=3276  OutDataTypeStr=Trq_Nm
  Asdrf_stInitin : Inport  Description=Status of Initialisation of ASD reference filter  Port=3  OutMin=0  OutMax=255  OutDataTypeStr=State_uint8
  Enable : EnablePort
  Add : Sum  Inputs=+-
  Bit Set : simulink/Logic and Bit Operations/Bit Set  iBit=2
  Bit Set1 : simulink/Logic and Bit Operations/Bit Set  iBit=3
  Bitwise Operator : simulink/Logic and Bit Operations/Bitwise Operator  logicop=OR  UseBitMask=off  NumInputPorts=2  BitMask=bin2dec('11011001')  BitMaskRealWorld=Stored Integer
  Constant : Constant  Value=0  OutDataTypeStr=Inherit: Inherit via back propagation
  Constant1 : Constant  Value=WESDem_stASDrfInit_C  OutMin=0  OutMax=255
  Data Store Read1 : DataStoreRead  DataStoreName=EISGov_st3
  Data Store Write1 : DataStoreWrite  DataStoreName=EISGov_st3
  MinMax : MinMax  Function=max  Inputs=2
  WESDem_trqReq : Outport  Tag=Nm  Description=Torque intialization request of working engine speed demand  OutMin=-3276  OutMax=3276  OutDataTypeStr=Trq_Nm
  asdrf_stInitOut : Outport  Port=2
  wires:
  Constant1/1 -> Bitwise Operator/2
  Asdrf_stInitin/1 -> Bitwise Operator/1
  PthSet_trqInrSet/1 -> Add/1
  CoETS_trqInrSetSlow/1 -> Add/2
  Add/1 -> MinMax/1
  Constant/1 -> MinMax/2
  MinMax/1 -> WESDem_trqReq/1
  Bitwise Operator/1 -> asdrf_stInitOut/1
  Data Store Read1/1 -> Bit Set/1
  Bit Set/1 -> Bit Set1/1
  Bit Set1/1 -> Data Store Write1/1

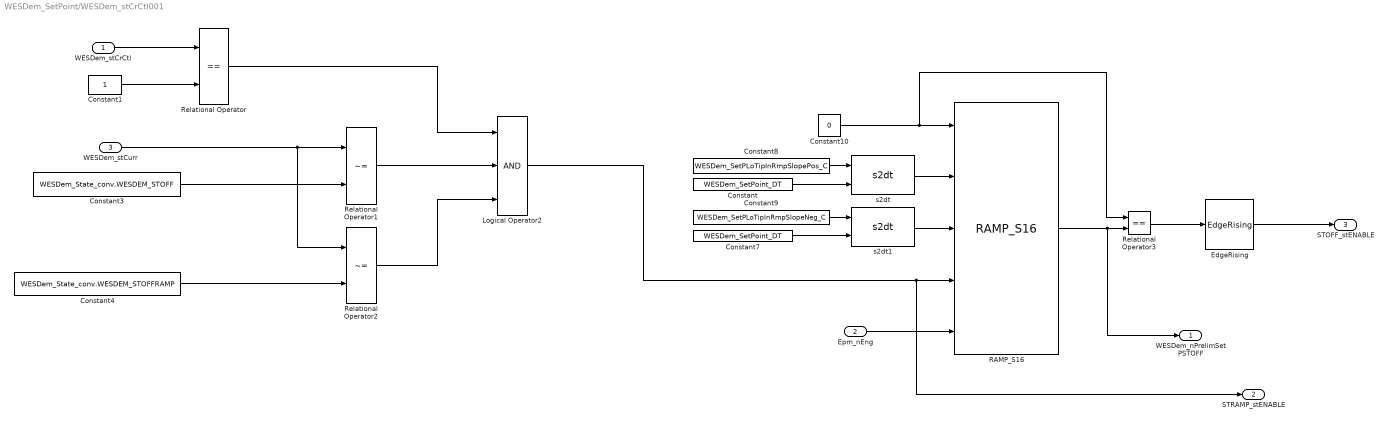
== system WESDem_SetPoint/WESDem_stCrCtl001 ==
  WESDem_stCrCtl : Inport  Description=State control of the working engine speed demand  OutMin=0  OutMax=65535  OutDataTypeStr=State_uint16
  Epm_nEng : Inport  Tag=rpm  Description=Engine speed  Port=2  OutMin=0  OutMax=6000  OutDataTypeStr=EngSpeed_rpm
  WESDem_stCurr : Inport  Port=3
  Constant : Constant  Value=WESDem_SetPoint_DT
  Constant1 : Constant  OutDataTypeStr=Inherit: Inherit via back propagation
  Constant10 : Constant  Value=0  OutDataTypeStr=Inherit: Inherit via back propagation
  Constant3 : Constant  Value=WESDem_State_conv.WESDEM_STOFF  OutDataTypeStr=Inherit: Inherit via back propagation
  Constant4 : Constant  Value=WESDem_State_conv.WESDEM_STOFFRAMP  OutDataTypeStr=Inherit: Inherit via back propagation
  Constant7 : Constant  Value=WESDem_SetPoint_DT
  Constant8 : Constant  Value=WESDem_SetPLoTipInRmpSlopePos_C
  Constant9 : Constant  Value=WESDem_SetPLoTipInRmpSlopeNeg_C
  EdgeRising : CXLib/EdgeRising
  Logical Operator2 : Logic  Inputs=3  AllPortsSameDT=off  OutDataTypeStr=boolean
  RAMP_S16 : CXLib/RAMP_S16
  Relational Operator : RelationalOperator  Operator===  OutDataTypeStr=boolean  RndMeth=Simplest
  Relational Operator1 : RelationalOperator  Operator=~=  OutDataTypeStr=boolean  RndMeth=Simplest
  Relational Operator2 : RelationalOperator  Operator=~=  OutDataTypeStr=boolean  RndMeth=Simplest
  Relational Operator3 : RelationalOperator  Operator===  OutDataTypeStr=boolean  RndMeth=Simplest
  s2dt : CXLib/s2dt
  s2dt1 : CXLib/s2dt
  WESDem_nPrelimSetPSTOFF : Outport
  STRAMP_stENABLE : Outport  Port=2
  STOFF_stENABLE : Outport  Port=3
  wires:
  WESDem_stCrCtl/1 -> Relational Operator/1
  Constant1/1 -> Relational Operator/2
  WESDem_stCurr/1 -> Relational Operator2/1, Relational Operator1/1
  Constant3/1 -> Relational Operator1/2
  Constant4/1 -> Relational Operator2/2
  Relational Operator1/1 -> Logical Operator2/2
  Relational Operator/1 -> Logical Operator2/1
  Relational Operator2/1 -> Logical Operator2/3
  Constant7/1 -> s2dt1/2
  s2dt/1 -> RAMP_S16/2
  Constant/1 -> s2dt/2
  Constant9/1 -> s2dt1/1
  Constant8/1 -> s2dt/1
  RAMP_S16/1 -> WESDem_nPrelimSetPSTOFF/1, Relational Operator3/2
  s2dt1/1 -> RAMP_S16/3
  Constant10/1 -> Relational Operator3/1, RAMP_S16/1
  Logical Operator2/1 -> STRAMP_stENABLE/1, RAMP_S16/4
  Epm_nEng/1 -> RAMP_S16/5
  Relational Operator3/1 -> EdgeRising/1
  EdgeRising/1 -> STOFF_stENABLE/1
